simulink model "current_fpga"  (R2020b)
settings: Solver=VariableStepAuto  StartTime=0.0  StopTime=10.0  RelTol=1e-3
settings Model: Creator=Student  LastModifiedBy=Student
settings OptimizationCC: BlockReduction=off  ConditionallyExecuteInputs=off  DefaultParameterBehavior=Inlined
settings DebuggingCC: AlgebraicLoopMsg=error
settings HardwareCC: ProdBitPerPointer=32  ProdBitPerSizeT=32  ProdBitPerPtrDiffT=32  ProdLargestAtomicFloat=None  ProdIntDivRoundTo=Undefined  ProdEndianess=Unspecified  ProdWordSize=32  ProdHWDeviceType=ASIC/FPGA->ASIC/FPGA  TargetBitPerPointer=64  TargetBitPerSizeT=64  TargetBitPerPtrDiffT=64  TargetLongLongMode=on  TargetIntDivRoundTo=Zero  TargetEndianess=LittleEndian  TargetWordSize=64  TargetHWDeviceType=Custom Processor->MATLAB Host Computer  ProdEqTarget=off

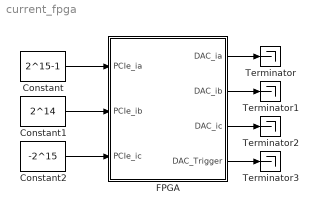
== system current_fpga ==
  Constant : Constant  Value=2^15-1  OutDataTypeStr=int16  SampleTime=5e-5
  Constant1 : Constant  Value=2^14  OutDataTypeStr=int16  SampleTime=5e-5
  Constant2 : Constant  Value=-2^15  OutDataTypeStr=int16  SampleTime=5e-5
  FPGA : Subsystem
  Terminator{,1..3} (4 alike) : Terminator
  wires:
  FPGA/1(DAC_ia) -> Terminator/1
  FPGA/4(DAC_Trigger) -> Terminator3/1
  FPGA/3(DAC_ic) -> Terminator2/1
  FPGA/2(DAC_ib) -> Terminator1/1
  Constant/1 -> FPGA/1(PCIe_ia)
  Constant2/1 -> FPGA/3(PCIe_ic)
  Constant1/1 -> FPGA/2(PCIe_ib)

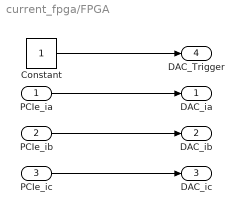
== system current_fpga/FPGA ==
  PCIe_ia : Inport
  PCIe_ib : Inport  Port=2
  PCIe_ic : Inport  Port=3
  Constant : Constant  OutDataTypeStr=boolean  SampleTime=-1
  DAC_ia : Outport
  DAC_ib : Outport  Port=2
  DAC_ic : Outport  Port=3
  DAC_Trigger : Outport  Port=4
  wires:
  PCIe_ic/1 -> DAC_ic/1
  PCIe_ib/1 -> DAC_ib/1
  PCIe_ia/1 -> DAC_ia/1
  Constant/1 -> DAC_Trigger/1
